simulink model "And2_Model"  (R2025a)
settings: Solver=VariableStepAuto  StartTime=0.0  StopTime=10.0  RelTol=1e-3
libraries: NSA_DEVS_SINKS x4, NSA_DEVS_SOURCES x2, NSA_DEVS_MATH_OPERATIONS x1, NSA_DEVS_LOGISTICS x1
settings Model: Creator=david  LastModifiedBy=peter
settings RTWCC: GPUComputeCapability=3.5

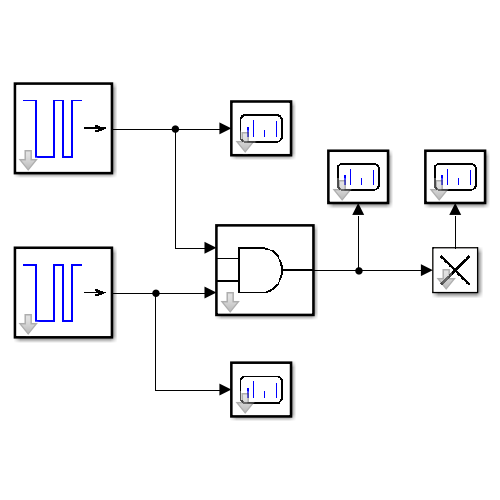
[thumbnail: Simulink's stored preview of the top-level diagram]
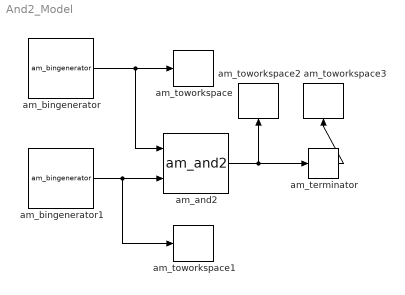
== system And2_Model ==
  am_and2 : NSA_DEVS_MATH_OPERATIONS/am_and2  i0=true  tau_copy=[0,1]  debug_copy=0
      settings: SourceProductName=Math Operations
  am_bingenerator : NSA_DEVS_SOURCES/am_bingenerator  z0=false  tVec=1:9  tau=[0,1]  debug=0
      settings: SourceProductName=Sources
  am_bingenerator1 : NSA_DEVS_SOURCES/am_bingenerator  z0=false  tVec=[1 3 5 7 100]  tau=[0,1]  debug=0
      settings: SourceProductName=Sources
  am_terminator : NSA_DEVS_LOGISTICS/am_terminator  countyEmptyInputs=false  tau_copy=[0,1]  debug_copy=0
      settings: SourceProductName=Logistics
  am_toworkspace : NSA_DEVS_SINKS/am_toworkspace  varname="\"gen1Out\""  t0=0  format="\"vector\""  tau=[0,5]  debug=0
      settings: SourceProductName=Sinks
  am_toworkspace1 : NSA_DEVS_SINKS/am_toworkspace  varname="\"gen2Out\""  t0=0  format="\"vector\""  tau=[0,5]  debug=0
      settings: SourceProductName=Sinks
  am_toworkspace2 : NSA_DEVS_SINKS/am_toworkspace  varname="\"andOut\""  t0=0  format="\"vector\""  tau=[0,5]  debug=0
      settings: SourceProductName=Sinks
  am_toworkspace3 : NSA_DEVS_SINKS/am_toworkspace  varname="\"nOut\""  t0=0  format="\"vector\""  tau=[0,5]  debug=0
      settings: SourceProductName=Sinks
  wires:
  am_bingenerator/1 -> am_and2/1, am_toworkspace/1
  am_and2/1 -> am_terminator/1, am_toworkspace2/1
  am_bingenerator1/1 -> am_and2/2, am_toworkspace1/1
  am_terminator/1 -> am_toworkspace3/1
